simulink model "HANcoder_E407_TTA_Template_DS_V2"  (R2023a)
settings: Solver=FixedStepDiscrete  StartTime=0.0  StopTime=1  FixedStep=0.01  RelTol=1e-3
PreLoadFcn:
  | librarySetup
  | eval([bdroot,'_startup']) %Calling [modelName]_startup.m
values from neighbouring files (symbols this model uses):
  basic_cycle_duration_bc0 = TM_Reset_Board   + COMP_duration    (= 372)    [HANcoder_E407_TTA_Template_DS_V1_startup.m]    (also in HANcoder_E407_TTA_Template_DS_V2_startup.m; HANcoder_E407_TTA_Template_DS_V52_startup.m; HANcoder_E407_TTA_Template_DS_V5_startup.m; HANcoder_E407_TTA_Template_DS_V6_startup.m = 532)
  basic_cycle_duration_bc1 = basic_cycle_duration_bc0    (= 372)    [HANcoder_E407_TTA_Template_DS_V1_startup.m]    (also in HANcoder_E407_TTA_Template_DS_V2_startup.m; HANcoder_E407_TTA_Template_DS_V52_startup.m; HANcoder_E407_TTA_Template_DS_V5_startup.m; HANcoder_E407_TTA_Template_DS_V6_startup.m = 532)
  basic_cycle_duration_bc2 = basic_cycle_duration_bc0    (= 372)    [HANcoder_E407_TTA_Template_DS_V1_startup.m]    (also in HANcoder_E407_TTA_Template_DS_V2_startup.m; HANcoder_E407_TTA_Template_DS_V52_startup.m; HANcoder_E407_TTA_Template_DS_V5_startup.m; HANcoder_E407_TTA_Template_DS_V6_startup.m = 532)
  comm_delay_estimation1 = round(comm_delay_measured1*hardware_granularity/frequency_IRQ)    [HANcoder_E407_TTA_Template_DS_V1_startup.m]    (also in HANcoder_E407_TTA_Template_DS_V2_startup.m; HANcoder_E407_TTA_Template_DS_V52_startup.m; HANcoder_E407_TTA_Template_DS_V5_startup.m; HANcoder_E407_TTA_Template_DS_V6_startup.m)
  comm_delay_estimation2 = round(comm_delay_measured2*hardware_granularity/frequency_IRQ)    [HANcoder_E407_TTA_Template_DS_V1_startup.m]    (also in HANcoder_E407_TTA_Template_DS_V2_startup.m; HANcoder_E407_TTA_Template_DS_V52_startup.m; HANcoder_E407_TTA_Template_DS_V5_startup.m; HANcoder_E407_TTA_Template_DS_V6_startup.m)
  COMM_Period = 80    [HANcoder_E407_TTA_Template_DS_V1_startup.m]    (also in HANcoder_E407_TTA_Template_DS_V2_startup.m; HANcoder_E407_TTA_Template_DS_V52_startup.m; HANcoder_E407_TTA_Template_DS_V5_startup.m; HANcoder_E407_TTA_Template_DS_V6_startup.m = 120)
  COMM_Phase1 = Simulink.Parameter    [HANcoder_E407_TTA_Template_DS_V1_startup.m]    (also in HANcoder_E407_TTA_Template_DS_V2_startup.m; HANcoder_E407_TTA_Template_DS_V52_startup.m; HANcoder_E407_TTA_Template_DS_V5_startup.m; HANcoder_E407_TTA_Template_DS_V6_startup.m)
  COMM_Phase2 = Simulink.Parameter    [HANcoder_E407_TTA_Template_DS_V1_startup.m]    (also in HANcoder_E407_TTA_Template_DS_V2_startup.m; HANcoder_E407_TTA_Template_DS_V52_startup.m; HANcoder_E407_TTA_Template_DS_V5_startup.m; HANcoder_E407_TTA_Template_DS_V6_startup.m)
  COMM_Phase_init1 = Simulink.Parameter    [HANcoder_E407_TTA_Template_DS_V1_startup.m]    (also in HANcoder_E407_TTA_Template_DS_V2_startup.m; HANcoder_E407_TTA_Template_DS_V52_startup.m; HANcoder_E407_TTA_Template_DS_V5_startup.m; HANcoder_E407_TTA_Template_DS_V6_startup.m)
  COMM_Phase_init2 = Simulink.Parameter    [HANcoder_E407_TTA_Template_DS_V1_startup.m]    (also in HANcoder_E407_TTA_Template_DS_V2_startup.m; HANcoder_E407_TTA_Template_DS_V52_startup.m; HANcoder_E407_TTA_Template_DS_V5_startup.m; HANcoder_E407_TTA_Template_DS_V6_startup.m)
  COMP_duration = 4    [HANcoder_E407_TTA_Template_DS_V1_startup.m]    (also in HANcoder_E407_TTA_Template_DS_V2_startup.m; HANcoder_E407_TTA_Template_DS_V52_startup.m; HANcoder_E407_TTA_Template_DS_V5_startup.m; HANcoder_E407_TTA_Template_DS_V6_startup.m)
  frequency_IRQ = 100    [HANcoder_E407_TTA_Template_DS_V1_startup.m]    (also in HANcoder_E407_TTA_Template_DS_V2_startup.m; HANcoder_E407_TTA_Template_DS_V52_startup.m; HANcoder_E407_TTA_Template_DS_V5_startup.m; HANcoder_E407_TTA_Template_DS_V6_startup.m)
  idle_time_init = basic_cycle_duration_bc0 + basic_cycle_duration_bc1    (= 744)    [HANcoder_E407_TTA_Template_DS_V1_startup.m]    (also in HANcoder_E407_TTA_Template_DS_V2_startup.m; HANcoder_E407_TTA_Template_DS_V52_startup.m = 1116; HANcoder_E407_TTA_Template_DS_V5_startup.m = 1116; HANcoder_E407_TTA_Template_DS_V6_startup.m = 1596)
  LA_Clock_Gr = 1    [HANcoder_E407_TTA_Template_DS_V1_startup.m]    (also in HANcoder_E407_TTA_Template_DS_V2_startup.m; HANcoder_E407_TTA_Template_DS_V52_startup.m; HANcoder_E407_TTA_Template_DS_V5_startup.m; HANcoder_E407_TTA_Template_DS_V6_startup.m)
  LA_COMM_dly = 1    [HANcoder_E407_TTA_Template_DS_V1_startup.m]    (also in HANcoder_E407_TTA_Template_DS_V2_startup.m; HANcoder_E407_TTA_Template_DS_V52_startup.m; HANcoder_E407_TTA_Template_DS_V5_startup.m; HANcoder_E407_TTA_Template_DS_V6_startup.m)
  LA_COMM_Err = 1    [HANcoder_E407_TTA_Template_DS_V1_startup.m]    (also in HANcoder_E407_TTA_Template_DS_V2_startup.m; HANcoder_E407_TTA_Template_DS_V52_startup.m; HANcoder_E407_TTA_Template_DS_V5_startup.m; HANcoder_E407_TTA_Template_DS_V6_startup.m)
  LA_E_Desync = 1    [HANcoder_E407_TTA_Template_DS_V1_startup.m]    (also in HANcoder_E407_TTA_Template_DS_V2_startup.m; HANcoder_E407_TTA_Template_DS_V52_startup.m; HANcoder_E407_TTA_Template_DS_V5_startup.m; HANcoder_E407_TTA_Template_DS_V6_startup.m)
  LA_MEX_Flag = 1    [HANcoder_E407_TTA_Template_DS_V1_startup.m]    (also in HANcoder_E407_TTA_Template_DS_V2_startup.m; HANcoder_E407_TTA_Template_DS_V52_startup.m; HANcoder_E407_TTA_Template_DS_V5_startup.m; HANcoder_E407_TTA_Template_DS_V6_startup.m)
  LA_Task_Act = 1    [HANcoder_E407_TTA_Template_DS_V1_startup.m]    (also in HANcoder_E407_TTA_Template_DS_V2_startup.m; HANcoder_E407_TTA_Template_DS_V52_startup.m; HANcoder_E407_TTA_Template_DS_V5_startup.m; HANcoder_E407_TTA_Template_DS_V6_startup.m)
  Master_Role = 1    [HANcoder_E407_TTA_Template_DS_V1_startup.m]    (also in HANcoder_E407_TTA_Template_DS_V2_startup.m; HANcoder_E407_TTA_Template_DS_V52_startup.m; HANcoder_E407_TTA_Template_DS_V5_startup.m; HANcoder_E407_TTA_Template_DS_V6_startup.m)
  matrix_rows = 3    [HANcoder_E407_TTA_Template_DS_V1_startup.m]    (also in HANcoder_E407_TTA_Template_DS_V2_startup.m; HANcoder_E407_TTA_Template_DS_V52_startup.m; HANcoder_E407_TTA_Template_DS_V5_startup.m; HANcoder_E407_TTA_Template_DS_V6_startup.m)
  max_desync = 15    [HANcoder_E407_TTA_Template_DS_V1_startup.m]    (also in HANcoder_E407_TTA_Template_DS_V2_startup.m; HANcoder_E407_TTA_Template_DS_V52_startup.m; HANcoder_E407_TTA_Template_DS_V5_startup.m; HANcoder_E407_TTA_Template_DS_V6_startup.m)
  max_num_msgs_CAN1 = 2^Tx_bit_number-1    (= 7)    [HANcoder_E407_TTA_Template_DS_V1_startup.m]    (also in HANcoder_E407_TTA_Template_DS_V2_startup.m; HANcoder_E407_TTA_Template_DS_V52_startup.m; HANcoder_E407_TTA_Template_DS_V5_startup.m; HANcoder_E407_TTA_Template_DS_V6_startup.m)
  max_num_msgs_CAN2 = max_num_msgs_CAN1    (= 7)    [HANcoder_E407_TTA_Template_DS_V1_startup.m]    (also in HANcoder_E407_TTA_Template_DS_V2_startup.m; HANcoder_E407_TTA_Template_DS_V52_startup.m; HANcoder_E407_TTA_Template_DS_V5_startup.m; HANcoder_E407_TTA_Template_DS_V6_startup.m)
  min_desync = (-1)*max_desync    (= -15)    [HANcoder_E407_TTA_Template_DS_V1_startup.m]    (also in HANcoder_E407_TTA_Template_DS_V2_startup.m; HANcoder_E407_TTA_Template_DS_V52_startup.m; HANcoder_E407_TTA_Template_DS_V5_startup.m; HANcoder_E407_TTA_Template_DS_V6_startup.m)
  PotValue1_ID = 22    [HANcoder_E407_TTA_Template_DS_V1_startup.m]    (also in HANcoder_E407_TTA_Template_DS_V2_startup.m; HANcoder_E407_TTA_Template_DS_V52_startup.m; HANcoder_E407_TTA_Template_DS_V5_startup.m; HANcoder_E407_TTA_Template_DS_V6_startup.m)
  PotValue2_ID = 23    [HANcoder_E407_TTA_Template_DS_V1_startup.m]    (also in HANcoder_E407_TTA_Template_DS_V2_startup.m; HANcoder_E407_TTA_Template_DS_V52_startup.m; HANcoder_E407_TTA_Template_DS_V5_startup.m; HANcoder_E407_TTA_Template_DS_V6_startup.m)
  PotValue3_ID = 24    [HANcoder_E407_TTA_Template_DS_V1_startup.m]    (also in HANcoder_E407_TTA_Template_DS_V2_startup.m; HANcoder_E407_TTA_Template_DS_V52_startup.m; HANcoder_E407_TTA_Template_DS_V5_startup.m; HANcoder_E407_TTA_Template_DS_V6_startup.m)
  script_run = Simulink.Parameter    [HANcoder_E407_TTA_Template_DS_V1_startup.m]    (also in HANcoder_E407_TTA_Template_DS_V2_startup.m; HANcoder_E407_TTA_Template_DS_V52_startup.m; HANcoder_E407_TTA_Template_DS_V5_startup.m; HANcoder_E407_TTA_Template_DS_V6_startup.m)
  Slave_Role = 2    [HANcoder_E407_TTA_Template_DS_V1_startup.m]    (also in HANcoder_E407_TTA_Template_DS_V2_startup.m; HANcoder_E407_TTA_Template_DS_V52_startup.m; HANcoder_E407_TTA_Template_DS_V5_startup.m; HANcoder_E407_TTA_Template_DS_V6_startup.m)
  Sync_ID = 1    [HANcoder_E407_TTA_Template_DS_V1_startup.m]    (also in HANcoder_E407_TTA_Template_DS_V2_startup.m; HANcoder_E407_TTA_Template_DS_V52_startup.m; HANcoder_E407_TTA_Template_DS_V5_startup.m; HANcoder_E407_TTA_Template_DS_V6_startup.m)
  TM_Check_PotValue1 = TM_COMM_PotValue1 + COMM_duration    (= 174)    [HANcoder_E407_TTA_Template_DS_V1_startup.m]    (also in HANcoder_E407_TTA_Template_DS_V2_startup.m; HANcoder_E407_TTA_Template_DS_V52_startup.m; HANcoder_E407_TTA_Template_DS_V5_startup.m; HANcoder_E407_TTA_Template_DS_V6_startup.m = 254)
  TM_Check_PotValue2 = TM_COMM_PotValue2 + COMM_duration    (= 258)    [HANcoder_E407_TTA_Template_DS_V1_startup.m]    (also in HANcoder_E407_TTA_Template_DS_V2_startup.m; HANcoder_E407_TTA_Template_DS_V52_startup.m; HANcoder_E407_TTA_Template_DS_V5_startup.m; HANcoder_E407_TTA_Template_DS_V6_startup.m = 378)
  TM_Check_PotValue3 = TM_COMM_PotValue3 + COMM_duration    (= 342)    [HANcoder_E407_TTA_Template_DS_V1_startup.m]    (also in HANcoder_E407_TTA_Template_DS_V2_startup.m; HANcoder_E407_TTA_Template_DS_V52_startup.m; HANcoder_E407_TTA_Template_DS_V5_startup.m; HANcoder_E407_TTA_Template_DS_V6_startup.m = 502)
  TM_Check_Sync = TM_COMM_Sync   + COMM_duration    (= 80)    [HANcoder_E407_TTA_Template_DS_V1_startup.m]    (also in HANcoder_E407_TTA_Template_DS_V2_startup.m; HANcoder_E407_TTA_Template_DS_V52_startup.m; HANcoder_E407_TTA_Template_DS_V5_startup.m; HANcoder_E407_TTA_Template_DS_V6_startup.m = 120)
  TM_Check_TOuts = TM_Count_Vote3 + COMP_duration    (= 356)    [HANcoder_E407_TTA_Template_DS_V1_startup.m]    (also in HANcoder_E407_TTA_Template_DS_V2_startup.m; HANcoder_E407_TTA_Template_DS_V52_startup.m; HANcoder_E407_TTA_Template_DS_V5_startup.m; HANcoder_E407_TTA_Template_DS_V6_startup.m = 516)
  TM_Check_Trailer1Articulation = TM_COMM_Trailer1Articulation + COMM_duration    (= 170)    [HANcoder_E407_TTA_Template_DS_V1_startup.m]    (also in HANcoder_E407_TTA_Template_DS_V2_startup.m; HANcoder_E407_TTA_Template_DS_V52_startup.m; HANcoder_E407_TTA_Template_DS_V5_startup.m; HANcoder_E407_TTA_Template_DS_V6_startup.m = 250)
  TM_Check_Trailer2Articulation = TM_COMM_Trailer2Articulation + COMM_duration    (= 254)    [HANcoder_E407_TTA_Template_DS_V1_startup.m]    (also in HANcoder_E407_TTA_Template_DS_V2_startup.m; HANcoder_E407_TTA_Template_DS_V52_startup.m; HANcoder_E407_TTA_Template_DS_V5_startup.m; HANcoder_E407_TTA_Template_DS_V6_startup.m = 374)
  TM_Check_Vote1 = TM_COMM_Vote1  + COMM_duration    (= 172)    [HANcoder_E407_TTA_Template_DS_V1_startup.m]    (also in HANcoder_E407_TTA_Template_DS_V2_startup.m; HANcoder_E407_TTA_Template_DS_V52_startup.m; HANcoder_E407_TTA_Template_DS_V5_startup.m; HANcoder_E407_TTA_Template_DS_V6_startup.m = 252)
  TM_Check_Vote2 = TM_COMM_Vote2  + COMM_duration    (= 260)    [HANcoder_E407_TTA_Template_DS_V1_startup.m]    (also in HANcoder_E407_TTA_Template_DS_V2_startup.m; HANcoder_E407_TTA_Template_DS_V52_startup.m; HANcoder_E407_TTA_Template_DS_V5_startup.m; HANcoder_E407_TTA_Template_DS_V6_startup.m = 380)
  TM_Check_Vote3 = TM_COMM_Vote3  + COMM_duration    (= 348)    [HANcoder_E407_TTA_Template_DS_V1_startup.m]    (also in HANcoder_E407_TTA_Template_DS_V2_startup.m; HANcoder_E407_TTA_Template_DS_V52_startup.m; HANcoder_E407_TTA_Template_DS_V5_startup.m; HANcoder_E407_TTA_Template_DS_V6_startup.m = 508)
  TM_COMM_PotValue1 = TM_ReadPot + COMP_duration    (= 94)    [HANcoder_E407_TTA_Template_DS_V1_startup.m]    (also in HANcoder_E407_TTA_Template_DS_V2_startup.m; HANcoder_E407_TTA_Template_DS_V52_startup.m; HANcoder_E407_TTA_Template_DS_V5_startup.m; HANcoder_E407_TTA_Template_DS_V6_startup.m = 134)
  TM_COMM_PotValue2 = TM_Check_PotValue1 + COMP_duration    (= 178)    [HANcoder_E407_TTA_Template_DS_V1_startup.m]    (also in HANcoder_E407_TTA_Template_DS_V2_startup.m; HANcoder_E407_TTA_Template_DS_V52_startup.m; HANcoder_E407_TTA_Template_DS_V5_startup.m; HANcoder_E407_TTA_Template_DS_V6_startup.m = 258)
  TM_COMM_PotValue3 = TM_Check_PotValue2 + COMP_duration    (= 262)    [HANcoder_E407_TTA_Template_DS_V1_startup.m]    (also in HANcoder_E407_TTA_Template_DS_V2_startup.m; HANcoder_E407_TTA_Template_DS_V52_startup.m; HANcoder_E407_TTA_Template_DS_V5_startup.m; HANcoder_E407_TTA_Template_DS_V6_startup.m = 382)
  TM_COMM_Sync = basic_cycle_start    (= 0)    [HANcoder_E407_TTA_Template_DS_V1_startup.m]    (also in HANcoder_E407_TTA_Template_DS_V2_startup.m; HANcoder_E407_TTA_Template_DS_V52_startup.m; HANcoder_E407_TTA_Template_DS_V5_startup.m; HANcoder_E407_TTA_Template_DS_V6_startup.m)
  TM_COMM_Trailer1Articulation = TM_Update_LT_2 + COMP_duration    (= 90)    [HANcoder_E407_TTA_Template_DS_V1_startup.m]    (also in HANcoder_E407_TTA_Template_DS_V2_startup.m; HANcoder_E407_TTA_Template_DS_V52_startup.m; HANcoder_E407_TTA_Template_DS_V5_startup.m; HANcoder_E407_TTA_Template_DS_V6_startup.m = 130)
  TM_COMM_Trailer2Articulation = TM_Check_Trailer1Articulation + COMP_duration    (= 174)    [HANcoder_E407_TTA_Template_DS_V1_startup.m]    (also in HANcoder_E407_TTA_Template_DS_V2_startup.m; HANcoder_E407_TTA_Template_DS_V52_startup.m; HANcoder_E407_TTA_Template_DS_V5_startup.m; HANcoder_E407_TTA_Template_DS_V6_startup.m = 254)
  TM_COMM_Vote1 = TM_Vote_Dec    + COMP_duration    (= 92)    [HANcoder_E407_TTA_Template_DS_V1_startup.m]    (also in HANcoder_E407_TTA_Template_DS_V2_startup.m; HANcoder_E407_TTA_Template_DS_V52_startup.m; HANcoder_E407_TTA_Template_DS_V5_startup.m; HANcoder_E407_TTA_Template_DS_V6_startup.m = 132)
  TM_COMM_Vote2 = TM_Count_Vote1 + COMP_duration    (= 180)    [HANcoder_E407_TTA_Template_DS_V1_startup.m]    (also in HANcoder_E407_TTA_Template_DS_V2_startup.m; HANcoder_E407_TTA_Template_DS_V52_startup.m; HANcoder_E407_TTA_Template_DS_V5_startup.m; HANcoder_E407_TTA_Template_DS_V6_startup.m = 260)
  TM_COMM_Vote3 = TM_Count_Vote2 + COMP_duration    (= 268)    [HANcoder_E407_TTA_Template_DS_V1_startup.m]    (also in HANcoder_E407_TTA_Template_DS_V2_startup.m; HANcoder_E407_TTA_Template_DS_V52_startup.m; HANcoder_E407_TTA_Template_DS_V5_startup.m; HANcoder_E407_TTA_Template_DS_V6_startup.m = 388)
  TM_Count_Vote1 = TM_Check_Vote1 + COMP_duration    (= 176)    [HANcoder_E407_TTA_Template_DS_V1_startup.m]    (also in HANcoder_E407_TTA_Template_DS_V2_startup.m; HANcoder_E407_TTA_Template_DS_V52_startup.m; HANcoder_E407_TTA_Template_DS_V5_startup.m; HANcoder_E407_TTA_Template_DS_V6_startup.m = 256)
  TM_Count_Vote2 = TM_Check_Vote2 + COMP_duration    (= 264)    [HANcoder_E407_TTA_Template_DS_V1_startup.m]    (also in HANcoder_E407_TTA_Template_DS_V2_startup.m; HANcoder_E407_TTA_Template_DS_V52_startup.m; HANcoder_E407_TTA_Template_DS_V5_startup.m; HANcoder_E407_TTA_Template_DS_V6_startup.m = 384)
  TM_Count_Vote3 = TM_Check_Vote3 + COMP_duration    (= 352)    [HANcoder_E407_TTA_Template_DS_V1_startup.m]    (also in HANcoder_E407_TTA_Template_DS_V2_startup.m; HANcoder_E407_TTA_Template_DS_V52_startup.m; HANcoder_E407_TTA_Template_DS_V5_startup.m; HANcoder_E407_TTA_Template_DS_V6_startup.m = 512)
  TM_Data_bc0 = TM_COMM_Sync    (= 0)    [HANcoder_E407_TTA_Template_DS_V1_startup.m]    (also in HANcoder_E407_TTA_Template_DS_V2_startup.m; HANcoder_E407_TTA_Template_DS_V52_startup.m; HANcoder_E407_TTA_Template_DS_V5_startup.m; HANcoder_E407_TTA_Template_DS_V6_startup.m)
  TM_Data_bc1 = TM_Data_bc0(1:4)    [HANcoder_E407_TTA_Template_DS_V1_startup.m]    (also in HANcoder_E407_TTA_Template_DS_V2_startup.m; HANcoder_E407_TTA_Template_DS_V52_startup.m; HANcoder_E407_TTA_Template_DS_V5_startup.m; HANcoder_E407_TTA_Template_DS_V6_startup.m)
  TM_Data_bc2 = TM_Data_bc0(1:4)    [HANcoder_E407_TTA_Template_DS_V1_startup.m]    (also in HANcoder_E407_TTA_Template_DS_V2_startup.m; HANcoder_E407_TTA_Template_DS_V52_startup.m; HANcoder_E407_TTA_Template_DS_V5_startup.m; HANcoder_E407_TTA_Template_DS_V6_startup.m)
  TM_New_Master = TM_Check_TOuts + COMP_duration    (= 360)    [HANcoder_E407_TTA_Template_DS_V1_startup.m]    (also in HANcoder_E407_TTA_Template_DS_V2_startup.m; HANcoder_E407_TTA_Template_DS_V52_startup.m; HANcoder_E407_TTA_Template_DS_V5_startup.m; HANcoder_E407_TTA_Template_DS_V6_startup.m = 520)
  TM_PotVote = TM_COMM_PotValue3 + COMP_duration    (= 266)    [HANcoder_E407_TTA_Template_DS_V1_startup.m]    (also in HANcoder_E407_TTA_Template_DS_V2_startup.m; HANcoder_E407_TTA_Template_DS_V52_startup.m; HANcoder_E407_TTA_Template_DS_V5_startup.m; HANcoder_E407_TTA_Template_DS_V6_startup.m = 386)
  TM_ReadPot = TM_Update_LT_2 + COMP_duration    (= 90)    [HANcoder_E407_TTA_Template_DS_V1_startup.m]    (also in HANcoder_E407_TTA_Template_DS_V2_startup.m; HANcoder_E407_TTA_Template_DS_V52_startup.m; HANcoder_E407_TTA_Template_DS_V5_startup.m; HANcoder_E407_TTA_Template_DS_V6_startup.m = 130)
  TM_Reset_Board = TM_Reset_Var   + COMP_duration    (= 368)    [HANcoder_E407_TTA_Template_DS_V1_startup.m]    (also in HANcoder_E407_TTA_Template_DS_V2_startup.m; HANcoder_E407_TTA_Template_DS_V52_startup.m; HANcoder_E407_TTA_Template_DS_V5_startup.m; HANcoder_E407_TTA_Template_DS_V6_startup.m = 528)
  TM_Reset_Var = TM_New_Master  + COMP_duration    (= 364)    [HANcoder_E407_TTA_Template_DS_V1_startup.m]    (also in HANcoder_E407_TTA_Template_DS_V2_startup.m; HANcoder_E407_TTA_Template_DS_V52_startup.m; HANcoder_E407_TTA_Template_DS_V5_startup.m; HANcoder_E407_TTA_Template_DS_V6_startup.m = 524)
  TM_Reset_Var_bc1 = TM_Data_bc1(end) + COMP_duration    [HANcoder_E407_TTA_Template_DS_V1_startup.m]    (also in HANcoder_E407_TTA_Template_DS_V2_startup.m; HANcoder_E407_TTA_Template_DS_V52_startup.m; HANcoder_E407_TTA_Template_DS_V5_startup.m; HANcoder_E407_TTA_Template_DS_V6_startup.m)
  TM_Reset_Var_bc1_2 = TM_Reset_Var_bc1 +2    [HANcoder_E407_TTA_Template_DS_V1_startup.m]    (also in HANcoder_E407_TTA_Template_DS_V2_startup.m; HANcoder_E407_TTA_Template_DS_V52_startup.m; HANcoder_E407_TTA_Template_DS_V5_startup.m; HANcoder_E407_TTA_Template_DS_V6_startup.m)
  TM_Type_bc0 = COMM    (= 0)    [HANcoder_E407_TTA_Template_DS_V1_startup.m]    (also in HANcoder_E407_TTA_Template_DS_V2_startup.m; HANcoder_E407_TTA_Template_DS_V52_startup.m; HANcoder_E407_TTA_Template_DS_V5_startup.m; HANcoder_E407_TTA_Template_DS_V6_startup.m)
  TM_Type_bc1 = TM_Type_bc0(1:4)    [HANcoder_E407_TTA_Template_DS_V1_startup.m]    (also in HANcoder_E407_TTA_Template_DS_V2_startup.m; HANcoder_E407_TTA_Template_DS_V52_startup.m; HANcoder_E407_TTA_Template_DS_V5_startup.m; HANcoder_E407_TTA_Template_DS_V6_startup.m)
  TM_Type_bc2 = TM_Type_bc0(1:4)    [HANcoder_E407_TTA_Template_DS_V1_startup.m]    (also in HANcoder_E407_TTA_Template_DS_V2_startup.m; HANcoder_E407_TTA_Template_DS_V52_startup.m; HANcoder_E407_TTA_Template_DS_V5_startup.m; HANcoder_E407_TTA_Template_DS_V6_startup.m)
  TM_Update_LT = TM_Check_Sync  + COMP_duration    (= 84)    [HANcoder_E407_TTA_Template_DS_V1_startup.m]    (also in HANcoder_E407_TTA_Template_DS_V2_startup.m; HANcoder_E407_TTA_Template_DS_V52_startup.m; HANcoder_E407_TTA_Template_DS_V5_startup.m; HANcoder_E407_TTA_Template_DS_V6_startup.m = 124)
  TM_Update_LT_2 = TM_Update_LT   + 2    (= 86)    [HANcoder_E407_TTA_Template_DS_V1_startup.m]    (also in HANcoder_E407_TTA_Template_DS_V2_startup.m; HANcoder_E407_TTA_Template_DS_V52_startup.m; HANcoder_E407_TTA_Template_DS_V5_startup.m; HANcoder_E407_TTA_Template_DS_V6_startup.m = 126)
  TM_Vote_Dec = TM_Update_LT   + COMP_duration    (= 88)    [HANcoder_E407_TTA_Template_DS_V1_startup.m]    (also in HANcoder_E407_TTA_Template_DS_V2_startup.m; HANcoder_E407_TTA_Template_DS_V52_startup.m; HANcoder_E407_TTA_Template_DS_V5_startup.m; HANcoder_E407_TTA_Template_DS_V6_startup.m = 128)
  Tractor_Board1 = 11    [HANcoder_E407_TTA_Template_DS_V1_startup.m]    (also in HANcoder_E407_TTA_Template_DS_V2_startup.m = 1; HANcoder_E407_TTA_Template_DS_V52_startup.m = 1; HANcoder_E407_TTA_Template_DS_V5_startup.m = 1; HANcoder_E407_TTA_Template_DS_V6_startup.m = 1)
  Tractor_Board2 = 12    [HANcoder_E407_TTA_Template_DS_V1_startup.m]    (also in HANcoder_E407_TTA_Template_DS_V2_startup.m = 2; HANcoder_E407_TTA_Template_DS_V52_startup.m = 2; HANcoder_E407_TTA_Template_DS_V5_startup.m = 2; HANcoder_E407_TTA_Template_DS_V6_startup.m = 2)
  Tractor_Board3 = 13    [HANcoder_E407_TTA_Template_DS_V1_startup.m]    (also in HANcoder_E407_TTA_Template_DS_V2_startup.m = 3; HANcoder_E407_TTA_Template_DS_V52_startup.m = 3; HANcoder_E407_TTA_Template_DS_V5_startup.m = 3; HANcoder_E407_TTA_Template_DS_V6_startup.m = 3)
  Trailer1_Articulation_ID = 31    [HANcoder_E407_TTA_Template_DS_V1_startup.m]    (also in HANcoder_E407_TTA_Template_DS_V2_startup.m; HANcoder_E407_TTA_Template_DS_V52_startup.m; HANcoder_E407_TTA_Template_DS_V5_startup.m; HANcoder_E407_TTA_Template_DS_V6_startup.m)
  Trailer1_Board1 = 2    [HANcoder_E407_TTA_Template_DS_V1_startup.m]    (also in HANcoder_E407_TTA_Template_DS_V2_startup.m = 4; HANcoder_E407_TTA_Template_DS_V52_startup.m = 4; HANcoder_E407_TTA_Template_DS_V5_startup.m = 4; HANcoder_E407_TTA_Template_DS_V6_startup.m = 4)
  Trailer1_Board2 = 3    [HANcoder_E407_TTA_Template_DS_V1_startup.m]    (also in HANcoder_E407_TTA_Template_DS_V2_startup.m = 5; HANcoder_E407_TTA_Template_DS_V52_startup.m = 5; HANcoder_E407_TTA_Template_DS_V5_startup.m = 5; HANcoder_E407_TTA_Template_DS_V6_startup.m = 5)
  Trailer1_Board3 = 4    [HANcoder_E407_TTA_Template_DS_V1_startup.m]    (also in HANcoder_E407_TTA_Template_DS_V2_startup.m = 6; HANcoder_E407_TTA_Template_DS_V52_startup.m = 6; HANcoder_E407_TTA_Template_DS_V5_startup.m = 6; HANcoder_E407_TTA_Template_DS_V6_startup.m = 6)
  Trailer2_Articulation_ID = 32    [HANcoder_E407_TTA_Template_DS_V1_startup.m]    (also in HANcoder_E407_TTA_Template_DS_V2_startup.m; HANcoder_E407_TTA_Template_DS_V52_startup.m; HANcoder_E407_TTA_Template_DS_V5_startup.m; HANcoder_E407_TTA_Template_DS_V6_startup.m)
  Trailer2_Board1 = 5    [HANcoder_E407_TTA_Template_DS_V1_startup.m]    (also in HANcoder_E407_TTA_Template_DS_V2_startup.m = 7; HANcoder_E407_TTA_Template_DS_V52_startup.m = 7; HANcoder_E407_TTA_Template_DS_V5_startup.m = 7; HANcoder_E407_TTA_Template_DS_V6_startup.m = 7)
  Trailer2_Board2 = 6    [HANcoder_E407_TTA_Template_DS_V1_startup.m]    (also in HANcoder_E407_TTA_Template_DS_V2_startup.m = 8; HANcoder_E407_TTA_Template_DS_V52_startup.m = 8; HANcoder_E407_TTA_Template_DS_V5_startup.m = 8; HANcoder_E407_TTA_Template_DS_V6_startup.m = 8)
  Trailer2_Board3 = 7    [HANcoder_E407_TTA_Template_DS_V1_startup.m]    (also in HANcoder_E407_TTA_Template_DS_V2_startup.m = 9; HANcoder_E407_TTA_Template_DS_V52_startup.m = 9; HANcoder_E407_TTA_Template_DS_V5_startup.m = 9; HANcoder_E407_TTA_Template_DS_V6_startup.m = 9)
  Vote1_ID = 11    [HANcoder_E407_TTA_Template_DS_V1_startup.m]    (also in HANcoder_E407_TTA_Template_DS_V2_startup.m; HANcoder_E407_TTA_Template_DS_V52_startup.m; HANcoder_E407_TTA_Template_DS_V5_startup.m; HANcoder_E407_TTA_Template_DS_V6_startup.m)
  Vote2_ID = 12    [HANcoder_E407_TTA_Template_DS_V1_startup.m]    (also in HANcoder_E407_TTA_Template_DS_V2_startup.m; HANcoder_E407_TTA_Template_DS_V52_startup.m; HANcoder_E407_TTA_Template_DS_V5_startup.m; HANcoder_E407_TTA_Template_DS_V6_startup.m)
  Vote3_ID = 13    [HANcoder_E407_TTA_Template_DS_V1_startup.m]    (also in HANcoder_E407_TTA_Template_DS_V2_startup.m; HANcoder_E407_TTA_Template_DS_V52_startup.m; HANcoder_E407_TTA_Template_DS_V5_startup.m; HANcoder_E407_TTA_Template_DS_V6_startup.m)
undefined symbols (not defined in the file or in its folder): A0, A1, A2, A3, A4, A5, CON2, CON4, D10, D12, D13, D8, D9
libraries: hdlsllib x160, HANcoder_STM32_Target x28, simulink x24, simulink_extras x1, dspstat3 x1
(part 34 of 35)

== system HANcoder_E407_TTA_Template_DS_V2/HANcoder STM32 Target - E407-STM32 algorithm/TTA CAN System/TTA System/Matrix Cycle Manager/Controller Matrix Cycle/controller basic cycle 2/COMP Task - Sync bc1 check/Process_Messages/Demux message CAN1 and check coherence/msg_count>2_DEBUG ==
  note: If this board received during this COMM a message
      | with a count greater than 1, it means the first message
      | sent was missed, but at least one later msg reached
      | this board.
  msg_c : Inport
  Constant : Constant
  Constant1 : Constant
  Data Store Read : DataStoreRead  DataStoreName=msg_count_DEBUG  IndexOptions=Index vector (dialog)  Indices=1  OutputSizes=1
  Data Store Read1 : DataStoreRead  DataStoreName=msg_count_DEBUG  IndexOptions=Index vector (dialog)  Indices=1  OutputSizes=1
  Data Store Write : DataStoreWrite  DataStoreName=msg_count_DEBUG  IndexOptions=Index vector (dialog)  Indices=1  OutputSizes=1
  GreaterThan : RelationalOperator  Operator=>  OutDataTypeStr=boolean  RndMeth=Simplest  InputSameDT=off
  Plus : Sum
  Switch : Switch  Criteria=u2 > Threshold  SaturateOnIntegerOverflow=off  InputSameDT=off
  wires:
  msg_c/1 -> GreaterThan/1
  Data Store Read/1 -> Switch/3
  Plus/1 -> Switch/1
  Data Store Read1/1 -> Plus/1
  Constant/1 -> Plus/2
  Switch/1 -> Data Store Write/1
  GreaterThan/1 -> Switch/2
  Constant1/1 -> GreaterThan/2

== system HANcoder_E407_TTA_Template_DS_V2/HANcoder STM32 Target - E407-STM32 algorithm/TTA CAN System/TTA System/Matrix Cycle Manager/Controller Matrix Cycle/controller basic cycle 2/COMP Task - Sync bc1 check/Process_Messages/Demux message CAN1 and check coherence1/Subsystem ==
  Msg_Temporal_Data : Inport
  Bit Shift : hdlsllib/Logic and Bit Operations/Bit Shift  mode=Shift Right Logical  N=7
  Bit Shift1 : hdlsllib/Logic and Bit Operations/Bit Shift  mode=Shift Right Logical  N=5
  Bit Shift2 : hdlsllib/Logic and Bit Operations/Bit Shift  mode=Shift Right Logical  N=4
  Bit Shift3 : hdlsllib/Logic and Bit Operations/Bit Shift  mode=Shift Left Logical  N=1
  Bit Shift4 : hdlsllib/Logic and Bit Operations/Bit Shift  mode=Shift Left Logical  N=4
  basic_cycle : Outport  VectorParamsAs1DForOutWhenUnconnected=off
  msg_count : Outport  Port=2  VectorParamsAs1DForOutWhenUnconnected=off
  board_id : Outport  Port=3  VectorParamsAs1DForOutWhenUnconnected=off
  wires:
  Bit Shift/1 -> basic_cycle/1
  Msg_Temporal_Data/1 -> Bit Shift4/1, Bit Shift/1, Bit Shift3/1
  Bit Shift1/1 -> msg_count/1
  Bit Shift2/1 -> board_id/1
  Bit Shift3/1 -> Bit Shift1/1
  Bit Shift4/1 -> Bit Shift2/1

== system HANcoder_E407_TTA_Template_DS_V2/HANcoder STM32 Target - E407-STM32 algorithm/TTA CAN System/TTA System/Matrix Cycle Manager/Controller Matrix Cycle/controller basic cycle 2/COMP Task - Sync bc1 check/Process_Messages/Demux message CAN1 and check coherence1/msg_count>2_DEBUG ==
  note: If this board received during this COMM a message
      | with a count greater than 1, it means the first message
      | sent was missed, but at least one later msg reached
      | this board.
  msg_c : Inport
  Constant : Constant
  Constant1 : Constant
  Data Store Read : DataStoreRead  DataStoreName=msg_count_DEBUG  IndexOptions=Index vector (dialog)  Indices=1  OutputSizes=1
  Data Store Read1 : DataStoreRead  DataStoreName=msg_count_DEBUG  IndexOptions=Index vector (dialog)  Indices=1  OutputSizes=1
  Data Store Write : DataStoreWrite  DataStoreName=msg_count_DEBUG  IndexOptions=Index vector (dialog)  Indices=1  OutputSizes=1
  GreaterThan : RelationalOperator  Operator=>  OutDataTypeStr=boolean  RndMeth=Simplest  InputSameDT=off
  Plus : Sum
  Switch : Switch  Criteria=u2 > Threshold  SaturateOnIntegerOverflow=off  InputSameDT=off
  wires:
  msg_c/1 -> GreaterThan/1
  Data Store Read/1 -> Switch/3
  Plus/1 -> Switch/1
  Data Store Read1/1 -> Plus/1
  Constant/1 -> Plus/2
  Switch/1 -> Data Store Write/1
  GreaterThan/1 -> Switch/2
  Constant1/1 -> GreaterThan/2

== system HANcoder_E407_TTA_Template_DS_V2/HANcoder STM32 Target - E407-STM32 algorithm/TTA CAN System/TTA System/Matrix Cycle Manager/Controller Matrix Cycle/controller basic cycle 0/COMM Task - Sync bc 0/Transmission subtasks/Check msg transmission CAN1/TX buffer update CAN1/Msg_Data_Encoder ==
  basic_cycle : Inport
  tx_counter : Inport  Port=2
  board_number : Inport  Port=3
  Bit Shift : hdlsllib/Logic and Bit Operations/Bit Shift  mode=Shift Left Logical  N=4
  Bit Shift1 : hdlsllib/Logic and Bit Operations/Bit Shift  mode=Shift Left Logical  N=7
  Minus : Sum  Inputs=3
  encoded_msg : Outport  VectorParamsAs1DForOutWhenUnconnected=off
  wires:
  basic_cycle/1 -> Bit Shift1/1
  Minus/1 -> encoded_msg/1
  tx_counter/1 -> Bit Shift/1
  Bit Shift1/1 -> Minus/1
  Bit Shift/1 -> Minus/2
  board_number/1 -> Minus/3

== system HANcoder_E407_TTA_Template_DS_V2/HANcoder STM32 Target - E407-STM32 algorithm/TTA CAN System/TTA System/Matrix Cycle Manager/Controller Matrix Cycle/controller basic cycle 0/COMM Task - Sync bc 0/Transmission subtasks/Check msg transmission CAN2/TX buffer update CAN2/Msg_Data_Encoder ==
  basic_cycle : Inport
  tx_counter : Inport  Port=2
  verif_value : Inport  Port=3
  Bit Shift : hdlsllib/Logic and Bit Operations/Bit Shift  mode=Shift Left Logical  N=4
  Bit Shift1 : hdlsllib/Logic and Bit Operations/Bit Shift  mode=Shift Left Logical  N=7
  Minus : Sum  Inputs=3
  encoded_msg : Outport  VectorParamsAs1DForOutWhenUnconnected=off
  wires:
  basic_cycle/1 -> Bit Shift1/1
  Minus/1 -> encoded_msg/1
  tx_counter/1 -> Bit Shift/1
  Bit Shift1/1 -> Minus/1
  Bit Shift/1 -> Minus/2
  verif_value/1 -> Minus/3

== system HANcoder_E407_TTA_Template_DS_V2/HANcoder STM32 Target - E407-STM32 algorithm/TTA CAN System/TTA System/Matrix Cycle Manager/Controller Matrix Cycle/controller basic cycle 0/COMM Task - Vote1/Transmission subtasks/Check msg transmission CAN1/TX buffer update CAN1/Msg_Data_Encoder ==
  basic_cycle : Inport
  tx_counter : Inport  Port=2
  board_number : Inport  Port=3
  Bit Shift : hdlsllib/Logic and Bit Operations/Bit Shift  mode=Shift Left Logical  N=4
  Bit Shift1 : hdlsllib/Logic and Bit Operations/Bit Shift  mode=Shift Left Logical  N=7
  Minus : Sum  Inputs=3
  encoded_msg : Outport  VectorParamsAs1DForOutWhenUnconnected=off
  wires:
  basic_cycle/1 -> Bit Shift1/1
  Minus/1 -> encoded_msg/1
  tx_counter/1 -> Bit Shift/1
  Bit Shift1/1 -> Minus/1
  Bit Shift/1 -> Minus/2
  board_number/1 -> Minus/3

== system HANcoder_E407_TTA_Template_DS_V2/HANcoder STM32 Target - E407-STM32 algorithm/TTA CAN System/TTA System/Matrix Cycle Manager/Controller Matrix Cycle/controller basic cycle 0/COMM Task - Vote1/Transmission subtasks/Check msg transmission CAN2/TX buffer update CAN2/Msg_Data_Encoder ==
  basic_cycle : Inport
  tx_counter : Inport  Port=2
  verif_value : Inport  Port=3
  Bit Shift : hdlsllib/Logic and Bit Operations/Bit Shift  mode=Shift Left Logical  N=4
  Bit Shift1 : hdlsllib/Logic and Bit Operations/Bit Shift  mode=Shift Left Logical  N=7
  Minus : Sum  Inputs=3
  encoded_msg : Outport  VectorParamsAs1DForOutWhenUnconnected=off
  wires:
  basic_cycle/1 -> Bit Shift1/1
  Minus/1 -> encoded_msg/1
  tx_counter/1 -> Bit Shift/1
  Bit Shift1/1 -> Minus/1
  Bit Shift/1 -> Minus/2
  verif_value/1 -> Minus/3

== system HANcoder_E407_TTA_Template_DS_V2/HANcoder STM32 Target - E407-STM32 algorithm/TTA CAN System/TTA System/Matrix Cycle Manager/Controller Matrix Cycle/controller basic cycle 0/COMM Task - Vote2/Transmission subtasks/Check msg transmission CAN1/TX buffer update CAN1/Msg_Data_Encoder ==
  basic_cycle : Inport
  tx_counter : Inport  Port=2
  board_number : Inport  Port=3
  Bit Shift : hdlsllib/Logic and Bit Operations/Bit Shift  mode=Shift Left Logical  N=4
  Bit Shift1 : hdlsllib/Logic and Bit Operations/Bit Shift  mode=Shift Left Logical  N=7
  Minus : Sum  Inputs=3
  encoded_msg : Outport  VectorParamsAs1DForOutWhenUnconnected=off
  wires:
  basic_cycle/1 -> Bit Shift1/1
  Minus/1 -> encoded_msg/1
  tx_counter/1 -> Bit Shift/1
  Bit Shift1/1 -> Minus/1
  Bit Shift/1 -> Minus/2
  board_number/1 -> Minus/3

== system HANcoder_E407_TTA_Template_DS_V2/HANcoder STM32 Target - E407-STM32 algorithm/TTA CAN System/TTA System/Matrix Cycle Manager/Controller Matrix Cycle/controller basic cycle 0/COMM Task - Vote2/Transmission subtasks/Check msg transmission CAN2/TX buffer update CAN2/Msg_Data_Encoder ==
  basic_cycle : Inport
  tx_counter : Inport  Port=2
  verif_value : Inport  Port=3
  Bit Shift : hdlsllib/Logic and Bit Operations/Bit Shift  mode=Shift Left Logical  N=4
  Bit Shift1 : hdlsllib/Logic and Bit Operations/Bit Shift  mode=Shift Left Logical  N=7
  Minus : Sum  Inputs=3
  encoded_msg : Outport  VectorParamsAs1DForOutWhenUnconnected=off
  wires:
  basic_cycle/1 -> Bit Shift1/1
  Minus/1 -> encoded_msg/1
  tx_counter/1 -> Bit Shift/1
  Bit Shift1/1 -> Minus/1
  Bit Shift/1 -> Minus/2
  verif_value/1 -> Minus/3

== system HANcoder_E407_TTA_Template_DS_V2/HANcoder STM32 Target - E407-STM32 algorithm/TTA CAN System/TTA System/Matrix Cycle Manager/Controller Matrix Cycle/controller basic cycle 0/COMM Task - Vote3/Transmission subtasks/Check msg transmission CAN1/TX buffer update CAN1/Msg_Data_Encoder ==
  basic_cycle : Inport
  tx_counter : Inport  Port=2
  board_number : Inport  Port=3
  Bit Shift : hdlsllib/Logic and Bit Operations/Bit Shift  mode=Shift Left Logical  N=4
  Bit Shift1 : hdlsllib/Logic and Bit Operations/Bit Shift  mode=Shift Left Logical  N=7
  Minus : Sum  Inputs=3
  encoded_msg : Outport  VectorParamsAs1DForOutWhenUnconnected=off
  wires:
  basic_cycle/1 -> Bit Shift1/1
  Minus/1 -> encoded_msg/1
  tx_counter/1 -> Bit Shift/1
  Bit Shift1/1 -> Minus/1
  Bit Shift/1 -> Minus/2
  board_number/1 -> Minus/3

== system HANcoder_E407_TTA_Template_DS_V2/HANcoder STM32 Target - E407-STM32 algorithm/TTA CAN System/TTA System/Matrix Cycle Manager/Controller Matrix Cycle/controller basic cycle 0/COMM Task - Vote3/Transmission subtasks/Check msg transmission CAN2/TX buffer update CAN2/Msg_Data_Encoder ==
  basic_cycle : Inport
  tx_counter : Inport  Port=2
  verif_value : Inport  Port=3
  Bit Shift : hdlsllib/Logic and Bit Operations/Bit Shift  mode=Shift Left Logical  N=4
  Bit Shift1 : hdlsllib/Logic and Bit Operations/Bit Shift  mode=Shift Left Logical  N=7
  Minus : Sum  Inputs=3
  encoded_msg : Outport  VectorParamsAs1DForOutWhenUnconnected=off
  wires:
  basic_cycle/1 -> Bit Shift1/1
  Minus/1 -> encoded_msg/1
  tx_counter/1 -> Bit Shift/1
  Bit Shift1/1 -> Minus/1
  Bit Shift/1 -> Minus/2
  verif_value/1 -> Minus/3

== system HANcoder_E407_TTA_Template_DS_V2/HANcoder STM32 Target - E407-STM32 algorithm/TTA CAN System/TTA System/Matrix Cycle Manager/Controller Matrix Cycle/controller basic cycle 1/COMM Task - PotValue trailer 1/Transmission subtasks/Check msg transmission CAN1/TX buffer update CAN1/Msg_Data_Encoder ==
  basic_cycle : Inport
  tx_counter : Inport  Port=2
  board_number : Inport  Port=3
  Bit Shift : hdlsllib/Logic and Bit Operations/Bit Shift  mode=Shift Left Logical  N=4
  Bit Shift1 : hdlsllib/Logic and Bit Operations/Bit Shift  mode=Shift Left Logical  N=7
  Minus : Sum  Inputs=3
  encoded_msg : Outport  VectorParamsAs1DForOutWhenUnconnected=off
  wires:
  basic_cycle/1 -> Bit Shift1/1
  Minus/1 -> encoded_msg/1
  tx_counter/1 -> Bit Shift/1
  Bit Shift1/1 -> Minus/1
  Bit Shift/1 -> Minus/2
  board_number/1 -> Minus/3

== system HANcoder_E407_TTA_Template_DS_V2/HANcoder STM32 Target - E407-STM32 algorithm/TTA CAN System/TTA System/Matrix Cycle Manager/Controller Matrix Cycle/controller basic cycle 1/COMM Task - PotValue trailer 1/Transmission subtasks/Check msg transmission CAN2/TX buffer update CAN2/Msg_Data_Encoder ==
  basic_cycle : Inport
  tx_counter : Inport  Port=2
  verif_value : Inport  Port=3
  Bit Shift : hdlsllib/Logic and Bit Operations/Bit Shift  mode=Shift Left Logical  N=4
  Bit Shift1 : hdlsllib/Logic and Bit Operations/Bit Shift  mode=Shift Left Logical  N=7
  Minus : Sum  Inputs=3
  encoded_msg : Outport  VectorParamsAs1DForOutWhenUnconnected=off
  wires:
  basic_cycle/1 -> Bit Shift1/1
  Minus/1 -> encoded_msg/1
  tx_counter/1 -> Bit Shift/1
  Bit Shift1/1 -> Minus/1
  Bit Shift/1 -> Minus/2
  verif_value/1 -> Minus/3

== system HANcoder_E407_TTA_Template_DS_V2/HANcoder STM32 Target - E407-STM32 algorithm/TTA CAN System/TTA System/Matrix Cycle Manager/Controller Matrix Cycle/controller basic cycle 1/COMM Task - PotValue trailer 2/Transmission subtasks/Check msg transmission CAN1/TX buffer update CAN1/Msg_Data_Encoder ==
  basic_cycle : Inport
  tx_counter : Inport  Port=2
  board_number : Inport  Port=3
  Bit Shift : hdlsllib/Logic and Bit Operations/Bit Shift  mode=Shift Left Logical  N=4
  Bit Shift1 : hdlsllib/Logic and Bit Operations/Bit Shift  mode=Shift Left Logical  N=7
  Minus : Sum  Inputs=3
  encoded_msg : Outport  VectorParamsAs1DForOutWhenUnconnected=off
  wires:
  basic_cycle/1 -> Bit Shift1/1
  Minus/1 -> encoded_msg/1
  tx_counter/1 -> Bit Shift/1
  Bit Shift1/1 -> Minus/1
  Bit Shift/1 -> Minus/2
  board_number/1 -> Minus/3

== system HANcoder_E407_TTA_Template_DS_V2/HANcoder STM32 Target - E407-STM32 algorithm/TTA CAN System/TTA System/Matrix Cycle Manager/Controller Matrix Cycle/controller basic cycle 1/COMM Task - PotValue trailer 2/Transmission subtasks/Check msg transmission CAN2/TX buffer update CAN2/Msg_Data_Encoder ==
  basic_cycle : Inport
  tx_counter : Inport  Port=2
  verif_value : Inport  Port=3
  Bit Shift : hdlsllib/Logic and Bit Operations/Bit Shift  mode=Shift Left Logical  N=4
  Bit Shift1 : hdlsllib/Logic and Bit Operations/Bit Shift  mode=Shift Left Logical  N=7
  Minus : Sum  Inputs=3
  encoded_msg : Outport  VectorParamsAs1DForOutWhenUnconnected=off
  wires:
  basic_cycle/1 -> Bit Shift1/1
  Minus/1 -> encoded_msg/1
  tx_counter/1 -> Bit Shift/1
  Bit Shift1/1 -> Minus/1
  Bit Shift/1 -> Minus/2
  verif_value/1 -> Minus/3

== system HANcoder_E407_TTA_Template_DS_V2/HANcoder STM32 Target - E407-STM32 algorithm/TTA CAN System/TTA System/Matrix Cycle Manager/Controller Matrix Cycle/controller basic cycle 1/COMM Task - PotValue trailer 3/Transmission subtasks/Check msg transmission CAN1/TX buffer update CAN1/Msg_Data_Encoder ==
  basic_cycle : Inport
  tx_counter : Inport  Port=2
  board_number : Inport  Port=3
  Bit Shift : hdlsllib/Logic and Bit Operations/Bit Shift  mode=Shift Left Logical  N=4
  Bit Shift1 : hdlsllib/Logic and Bit Operations/Bit Shift  mode=Shift Left Logical  N=7
  Minus : Sum  Inputs=3
  encoded_msg : Outport  VectorParamsAs1DForOutWhenUnconnected=off
  wires:
  basic_cycle/1 -> Bit Shift1/1
  Minus/1 -> encoded_msg/1
  tx_counter/1 -> Bit Shift/1
  Bit Shift1/1 -> Minus/1
  Bit Shift/1 -> Minus/2
  board_number/1 -> Minus/3

== system HANcoder_E407_TTA_Template_DS_V2/HANcoder STM32 Target - E407-STM32 algorithm/TTA CAN System/TTA System/Matrix Cycle Manager/Controller Matrix Cycle/controller basic cycle 1/COMM Task - PotValue trailer 3/Transmission subtasks/Check msg transmission CAN2/TX buffer update CAN2/Msg_Data_Encoder ==
  basic_cycle : Inport
  tx_counter : Inport  Port=2
  verif_value : Inport  Port=3
  Bit Shift : hdlsllib/Logic and Bit Operations/Bit Shift  mode=Shift Left Logical  N=4
  Bit Shift1 : hdlsllib/Logic and Bit Operations/Bit Shift  mode=Shift Left Logical  N=7
  Minus : Sum  Inputs=3
  encoded_msg : Outport  VectorParamsAs1DForOutWhenUnconnected=off
  wires:
  basic_cycle/1 -> Bit Shift1/1
  Minus/1 -> encoded_msg/1
  tx_counter/1 -> Bit Shift/1
  Bit Shift1/1 -> Minus/1
  Bit Shift/1 -> Minus/2
  verif_value/1 -> Minus/3

== system HANcoder_E407_TTA_Template_DS_V2/HANcoder STM32 Target - E407-STM32 algorithm/TTA CAN System/TTA System/Matrix Cycle Manager/Controller Matrix Cycle/controller basic cycle 1/COMM Task - Sync bc 1/Transmission subtasks1/Check msg transmission CAN1/TX buffer update CAN1/Msg_Data_Encoder ==
  basic_cycle : Inport
  tx_counter : Inport  Port=2
  board_number : Inport  Port=3
  Bit Shift : hdlsllib/Logic and Bit Operations/Bit Shift  mode=Shift Left Logical  N=4
  Bit Shift1 : hdlsllib/Logic and Bit Operations/Bit Shift  mode=Shift Left Logical  N=7
  Minus : Sum  Inputs=3
  encoded_msg : Outport  VectorParamsAs1DForOutWhenUnconnected=off
  wires:
  basic_cycle/1 -> Bit Shift1/1
  Minus/1 -> encoded_msg/1
  tx_counter/1 -> Bit Shift/1
  Bit Shift1/1 -> Minus/1
  Bit Shift/1 -> Minus/2
  board_number/1 -> Minus/3

== system HANcoder_E407_TTA_Template_DS_V2/HANcoder STM32 Target - E407-STM32 algorithm/TTA CAN System/TTA System/Matrix Cycle Manager/Controller Matrix Cycle/controller basic cycle 1/COMM Task - Sync bc 1/Transmission subtasks1/Check msg transmission CAN2/TX buffer update CAN2/Msg_Data_Encoder ==
  basic_cycle : Inport
  tx_counter : Inport  Port=2
  verif_value : Inport  Port=3
  Bit Shift : hdlsllib/Logic and Bit Operations/Bit Shift  mode=Shift Left Logical  N=4
  Bit Shift1 : hdlsllib/Logic and Bit Operations/Bit Shift  mode=Shift Left Logical  N=7
  Minus : Sum  Inputs=3
  encoded_msg : Outport  VectorParamsAs1DForOutWhenUnconnected=off
  wires:
  basic_cycle/1 -> Bit Shift1/1
  Minus/1 -> encoded_msg/1
  tx_counter/1 -> Bit Shift/1
  Bit Shift1/1 -> Minus/1
  Bit Shift/1 -> Minus/2
  verif_value/1 -> Minus/3

== system HANcoder_E407_TTA_Template_DS_V2/HANcoder STM32 Target - E407-STM32 algorithm/TTA CAN System/TTA System/Matrix Cycle Manager/Controller Matrix Cycle/controller basic cycle 2/COMM Task - Articualtion angle trailer 1/Transmission subtasks/Check msg transmission CAN1/TX buffer update CAN1/Msg_Data_Encoder1 ==
  basic_cycle : Inport
  tx_counter : Inport  Port=2
  board_number : Inport  Port=3
  Bit Concat : hdlsllib/Logic and Bit Operations/Bit Concat  numInputs=3
  Extract Bits : simulink/Logic and Bit Operations/Extract Bits  bitsToExtract=Range ending with least significant bit  numBits=2  bitIdxRange=[0 7]  outScalingMode=Treat bit field as an integer
  Extract Bits1 : simulink/Logic and Bit Operations/Extract Bits  bitsToExtract=Range ending with least significant bit  numBits=2  bitIdxRange=[0 7]  outScalingMode=Treat bit field as an integer
  Extract Bits2 : simulink/Logic and Bit Operations/Extract Bits  bitsToExtract=Range ending with least significant bit  numBits=4  bitIdxRange=[0 7]  outScalingMode=Treat bit field as an integer
  encoded_msg : Outport  VectorParamsAs1DForOutWhenUnconnected=off
  wires:
  Bit Concat/1 -> encoded_msg/1
  Extract Bits/1 -> Bit Concat/1
  Extract Bits1/1 -> Bit Concat/2
  Extract Bits2/1 -> Bit Concat/3
  basic_cycle/1 -> Extract Bits/1
  tx_counter/1 -> Extract Bits1/1
  board_number/1 -> Extract Bits2/1

== system HANcoder_E407_TTA_Template_DS_V2/HANcoder STM32 Target - E407-STM32 algorithm/TTA CAN System/TTA System/Matrix Cycle Manager/Controller Matrix Cycle/controller basic cycle 2/COMM Task - Articualtion angle trailer 1/Transmission subtasks/Check msg transmission CAN2/TX buffer update CAN2/Msg_Data_Encoder1 ==
  basic_cycle : Inport
  tx_counter : Inport  Port=2
  board_number : Inport  Port=3
  Bit Concat : hdlsllib/Logic and Bit Operations/Bit Concat  numInputs=3
  Extract Bits : simulink/Logic and Bit Operations/Extract Bits  bitsToExtract=Range ending with least significant bit  numBits=2  bitIdxRange=[0 7]  outScalingMode=Treat bit field as an integer
  Extract Bits1 : simulink/Logic and Bit Operations/Extract Bits  bitsToExtract=Range ending with least significant bit  numBits=2  bitIdxRange=[0 7]  outScalingMode=Treat bit field as an integer
  Extract Bits2 : simulink/Logic and Bit Operations/Extract Bits  bitsToExtract=Range ending with least significant bit  numBits=4  bitIdxRange=[0 7]  outScalingMode=Treat bit field as an integer
  encoded_msg : Outport  VectorParamsAs1DForOutWhenUnconnected=off
  wires:
  Bit Concat/1 -> encoded_msg/1
  Extract Bits/1 -> Bit Concat/1
  Extract Bits1/1 -> Bit Concat/2
  Extract Bits2/1 -> Bit Concat/3
  basic_cycle/1 -> Extract Bits/1
  tx_counter/1 -> Extract Bits1/1
  board_number/1 -> Extract Bits2/1

== system HANcoder_E407_TTA_Template_DS_V2/HANcoder STM32 Target - E407-STM32 algorithm/TTA CAN System/TTA System/Matrix Cycle Manager/Controller Matrix Cycle/controller basic cycle 2/COMM Task - Articualtion angle trailer 2/Transmission subtasks/Check msg transmission CAN1/TX buffer update CAN1/Msg_Data_Encoder1 ==
  basic_cycle : Inport
  tx_counter : Inport  Port=2
  board_number : Inport  Port=3
  Bit Concat : hdlsllib/Logic and Bit Operations/Bit Concat  numInputs=3
  Extract Bits : simulink/Logic and Bit Operations/Extract Bits  bitsToExtract=Range ending with least significant bit  numBits=2  bitIdxRange=[0 7]  outScalingMode=Treat bit field as an integer
  Extract Bits1 : simulink/Logic and Bit Operations/Extract Bits  bitsToExtract=Range ending with least significant bit  numBits=2  bitIdxRange=[0 7]  outScalingMode=Treat bit field as an integer
  Extract Bits2 : simulink/Logic and Bit Operations/Extract Bits  bitsToExtract=Range ending with least significant bit  numBits=4  bitIdxRange=[0 7]  outScalingMode=Treat bit field as an integer
  encoded_msg : Outport  VectorParamsAs1DForOutWhenUnconnected=off
  wires:
  Bit Concat/1 -> encoded_msg/1
  Extract Bits/1 -> Bit Concat/1
  Extract Bits1/1 -> Bit Concat/2
  Extract Bits2/1 -> Bit Concat/3
  basic_cycle/1 -> Extract Bits/1
  tx_counter/1 -> Extract Bits1/1
  board_number/1 -> Extract Bits2/1

== system HANcoder_E407_TTA_Template_DS_V2/HANcoder STM32 Target - E407-STM32 algorithm/TTA CAN System/TTA System/Matrix Cycle Manager/Controller Matrix Cycle/controller basic cycle 2/COMM Task - Articualtion angle trailer 2/Transmission subtasks/Check msg transmission CAN2/TX buffer update CAN2/Msg_Data_Encoder1 ==
  basic_cycle : Inport
  tx_counter : Inport  Port=2
  board_number : Inport  Port=3
  Bit Concat : hdlsllib/Logic and Bit Operations/Bit Concat  numInputs=3
  Extract Bits : simulink/Logic and Bit Operations/Extract Bits  bitsToExtract=Range ending with least significant bit  numBits=2  bitIdxRange=[0 7]  outScalingMode=Treat bit field as an integer
  Extract Bits1 : simulink/Logic and Bit Operations/Extract Bits  bitsToExtract=Range ending with least significant bit  numBits=2  bitIdxRange=[0 7]  outScalingMode=Treat bit field as an integer
  Extract Bits2 : simulink/Logic and Bit Operations/Extract Bits  bitsToExtract=Range ending with least significant bit  numBits=4  bitIdxRange=[0 7]  outScalingMode=Treat bit field as an integer
  encoded_msg : Outport  VectorParamsAs1DForOutWhenUnconnected=off
  wires:
  Bit Concat/1 -> encoded_msg/1
  Extract Bits/1 -> Bit Concat/1
  Extract Bits1/1 -> Bit Concat/2
  Extract Bits2/1 -> Bit Concat/3
  basic_cycle/1 -> Extract Bits/1
  tx_counter/1 -> Extract Bits1/1
  board_number/1 -> Extract Bits2/1

== system HANcoder_E407_TTA_Template_DS_V2/HANcoder STM32 Target - E407-STM32 algorithm/TTA CAN System/TTA System/Matrix Cycle Manager/Controller Matrix Cycle/controller basic cycle 2/COMM Task - Sync bc 1/Transmission subtasks1/Check msg transmission CAN1/TX buffer update CAN1/Msg_Data_Encoder ==
  basic_cycle : Inport
  tx_counter : Inport  Port=2
  board_number : Inport  Port=3
  Bit Shift : hdlsllib/Logic and Bit Operations/Bit Shift  mode=Shift Left Logical  N=4
  Bit Shift1 : hdlsllib/Logic and Bit Operations/Bit Shift  mode=Shift Left Logical  N=7
  Minus : Sum  Inputs=3
  encoded_msg : Outport  VectorParamsAs1DForOutWhenUnconnected=off
  wires:
  basic_cycle/1 -> Bit Shift1/1
  Minus/1 -> encoded_msg/1
  tx_counter/1 -> Bit Shift/1
  Bit Shift1/1 -> Minus/1
  Bit Shift/1 -> Minus/2
  board_number/1 -> Minus/3

== system HANcoder_E407_TTA_Template_DS_V2/HANcoder STM32 Target - E407-STM32 algorithm/TTA CAN System/TTA System/Matrix Cycle Manager/Controller Matrix Cycle/controller basic cycle 2/COMM Task - Sync bc 1/Transmission subtasks1/Check msg transmission CAN2/TX buffer update CAN2/Msg_Data_Encoder ==
  basic_cycle : Inport
  tx_counter : Inport  Port=2
  verif_value : Inport  Port=3
  Bit Shift : hdlsllib/Logic and Bit Operations/Bit Shift  mode=Shift Left Logical  N=4
  Bit Shift1 : hdlsllib/Logic and Bit Operations/Bit Shift  mode=Shift Left Logical  N=7
  Minus : Sum  Inputs=3
  encoded_msg : Outport  VectorParamsAs1DForOutWhenUnconnected=off
  wires:
  basic_cycle/1 -> Bit Shift1/1
  Minus/1 -> encoded_msg/1
  tx_counter/1 -> Bit Shift/1
  Bit Shift1/1 -> Minus/1
  Bit Shift/1 -> Minus/2
  verif_value/1 -> Minus/3

== matlab function HANcoder_E407_TTA_Template_DS_V2/HANcoder STM32 Target - E407-STM32 algorithm/TTA CAN System/TTA System/Matrix Cycle Manager/Controller Matrix Cycle/controller basic cycle 1/COMP Task - Potentiometer Voting/MATLAB Function ==
  data: u1 input; y output; u2 input; u3 input
function y = fcn(u1,u2,u3)

if (u1 == 1) && (u2 == 1) && (u3 == 1)

    y = 0;

elseif (u1 == 1) && (u2 == 0) && (u3 == 0)
    y = 3;

elseif (u1 == 0) && (u2 == 1) && (u3 == 0)
    y = 1;

elseif (u1 == 0) && (u2 == 0) && (u3 == 1)
    y = 2;

else 
    y = 0;
end
